simulink model "MC_HEXA_MISSION"  (R2023b)
settings: Solver=FixedStepDiscrete  StartTime=0.0  StopTime=inf  FixedStep=1/250  RelTol=1e-3  EnableMultiTasking=on
values from neighbouring files (symbols this model uses):
  SampleTime = 1/250    (= 0.004)    [Init_FLIGHT_Hexacopter.m]    (also in Init_FLIGHT_Hexacopter_fromNCMS.m = 0.01)
undefined symbols (not defined in the file or in its folder): control, IDLEPWM, MC_PITCH_P, MC_PITCHRATE_D, MC_PITCHRATE_I, MC_PITCHRATE_P, MC_ROLL_P, MC_ROLLRATE_D, MC_ROLLRATE_I, MC_ROLLRATE_P, MC_YAW_P, MC_YAWRATE_D, MC_YAWRATE_I, MC_YAWRATE_P, MPC_XY_P, MPC_XY_VEL_MAX, MPC_Z_D, MPC_Z_I, MPC_Z_P, MPC_Z_VEL_D_ACC, MPC_Z_VEL_I_ACC, MPC_Z_VEL_MAX_DN, MPC_Z_VEL_MAX_UP, MPC_Z_VEL_P_ACC, noutputs, output, pitch, pitch_body, roll, roll_body, TargetHardware, thrust_body, timestamp, x, y, yaw, yaw_body, z
libraries: px4lib x45, px4uORBlib x19, slpidlib x10, simulink x9, px4Utilslib x5, simulink_extras x5, uavalgslib x3, px4Sensorslib x2, sharedutil x1, sharedtransform x1
(part 1 of 4)
settings Model: ExtModeTrigDuration=10  Creator=The MathWorks, Inc.  LastModifiedBy=UASG
settings SolverCC: PositivePriorityOrder=on  MaxZcPerStep=1
settings OptimizationCC: DefaultUnderspecifiedDataType=single  StrengthReduction=on  PassReuseOutputArgsAs=Individual arguments  ZeroExternalMemoryAtStartup=off  ZeroInternalMemoryAtStartup=off  MaxStackSize=64  OptimizeBlockOrder=speed  OptimizationPriority=Speed  OptimizationCustomize=off  MultiThreadedLoops=on  EfficientTunableParamExpr=on
settings DebuggingCC: ParameterTunabilityLossMsg=error
settings HardwareCC: ProdBitPerPointer=32  ProdBitPerSizeT=32  ProdBitPerPtrDiffT=32  ProdLargestAtomicInteger=Long  ProdLargestAtomicFloat=Double  ProdWordSize=32  ProdLongLongMode=on  ProdHWDeviceType=ARM Compatible->ARM Cortex
settings ModelReferenceCC: EnableRefExpFcnMdlSchedulingChecks=on
settings SFSimCC: MATLABDynamicMemAlloc=off  SimTargetLang=C++
settings RTWCC: Description=Embedded Coder  SystemTargetFile=ert.tlc  HardwareBoard=PX4 Cube Orange  TLCOptions="-aInlineSetEventsForThisBaseRateFcn=TLC_FALSE -aSuppressMultiTaskScheduler=TLC_FALSE  -aRateBasedStepFcn=0"  TemplateMakefile=ert_default_tmf  GenerateReport=on  Toolchain=GNU Tools for PX4 Autopilots  BuildConfiguration=Faster Runs  LaunchReport=on  TargetLang=C++  DLArmComputeVersion=19.05
settings CodeAppCC: ForceParamTrailComments=on  IgnoreCustomStorageClasses=off  MaxIdLength=63  OperatorAnnotations=on  SimulinkDataObjDesc=on  SFDataObjDesc=on  InsertBlockDesc=on
settings ERTTargetCC: ExtModeTransport=3  ExtModeStaticAlloc=on  ExtModeStaticAllocSize=1024  ExtModeMexFile=ext_xcp  ExtModeIntrfLevel=Level2 - Open

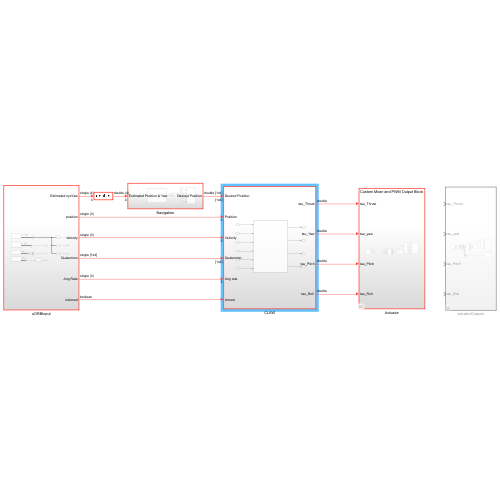
[thumbnail: Simulink's stored preview of the top-level diagram]
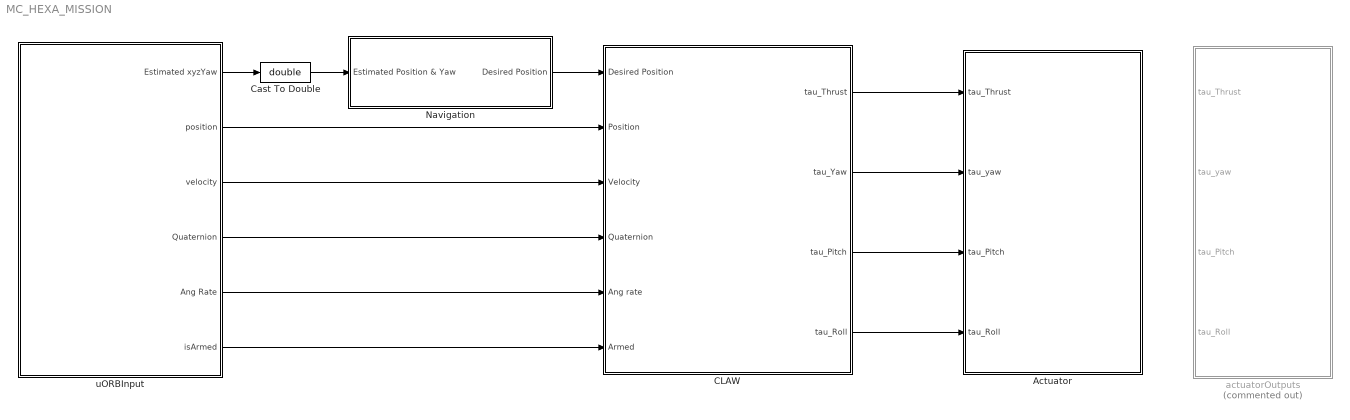
== system MC_HEXA_MISSION ==
  Actuator : Subsystem  Variant=on
  CLAW : Subsystem  RTWFcnName=CLAW
      settings: RTWSystemCode=Nonreusable function  RTWFcnNameOpts=Use subsystem name  RTWFileNameOpts=Use subsystem name
  Cast To Double : DataTypeConversion  OutDataTypeStr=double  SaturateOnIntegerOverflow=off  RndMeth=Floor
  Navigation : Subsystem
      settings: RTWSystemCode=Nonreusable function  RTWFcnNameOpts=Use subsystem name  RTWFileNameOpts=Use subsystem name
  actuatorOutputs : Subsystem  Commented=on  TreatAsAtomicUnit=on
      settings: RTWSystemCode=Nonreusable function  RTWFcnNameOpts=Use subsystem name  RTWFileNameOpts=Use subsystem name
  uORBInput : Subsystem
      settings: RTWSystemCode=Nonreusable function  RTWFcnNameOpts=Use subsystem name  RTWFileNameOpts=Use subsystem name
  wires:
  Navigation/1(Desired Position) -> CLAW/1(Desired Position)
  uORBInput/1(Estimated xyzYaw) -> Cast To Double/1
  uORBInput/3(velocity) -> CLAW/3(Velocity)
  uORBInput/4(Quaternion) -> CLAW/4(Quaternion)
  uORBInput/5(Ang Rate) -> CLAW/5(Ang rate)
  uORBInput/6(isArmed) -> CLAW/6(Armed)
  uORBInput/2(position) -> CLAW/2(Position)
  CLAW/1(tau_Thrust) -> Actuator/1(tau_Thrust)
  CLAW/3(tau_Pitch) -> Actuator/3(tau_Pitch)
  CLAW/2(tau_Yaw) -> Actuator/2(tau_yaw)
  CLAW/4("tau_Roll ") -> Actuator/4(tau_Roll)
  Cast To Double/1 -> Navigation/1(Estimated Position & Yaw)

== system MC_HEXA_MISSION/Actuator ==
  tau_Thrust : Inport
  tau_yaw : Inport  Port=2
  tau_Pitch : Inport  Port=3
  tau_Roll : Inport  Port=4
  Custom Mixer and PWM Output Block : Subsystem  VariantControl=useCustomMixer == true
  PX4 Mixer and actuator_controls_0 topic : Subsystem  VariantControl=useCustomMixer == false

== system MC_HEXA_MISSION/CLAW ==
  Desired Position : Inport
  Position : Inport  Port=2
  Velocity : Inport  Port=3
  Quaternion : Inport  Port=4
  Ang rate : Inport  Port=5
  Armed : Inport  Port=6
  Controller : Subsystem
  tau_Thrust : Outport
  tau_Yaw : Outport  Port=2
  tau_Pitch : Outport  Port=3
  "tau_Roll " : Outport  Port=4
  wires:
  Controller/3(tau_Pitch) -> tau_Pitch/1
  Controller/2(tau_Yaw) -> tau_Yaw/1
  Controller/4("tau_Roll ") -> "tau_Roll "/1
  Controller/1(tau_Thrust) -> tau_Thrust/1
  Desired Position/1 -> Controller/5(Desired Position)
  Position/1 -> Controller/1(Position)
  Velocity/1 -> Controller/2(Velocity)
  Quaternion/1 -> Controller/3(Quaternion)
  Ang rate/1 -> Controller/4(Ang rate)
  Armed/1 -> Controller/6(Armed)

== system MC_HEXA_MISSION/Navigation ==
  Estimated Position & Yaw : Inport
  Demux : Demux
  Quadcopter Navigation Algorithm : Subsystem  Variant=on
  uORB Publish : Subsystem
  Desired Position : Outport
  wires:
  Quadcopter Navigation Algorithm/1(Desired Position) -> Demux/1, Desired Position/1
  Estimated Position & Yaw/1 -> Quadcopter Navigation Algorithm/1(Current Position)
  Demux/1 -> uORB Publish/1(x_sp)
  Demux/2 -> uORB Publish/2(y_sp)
  Demux/3 -> uORB Publish/3(z_sp)
  Demux/4 -> uORB Publish/4(heading_sp)

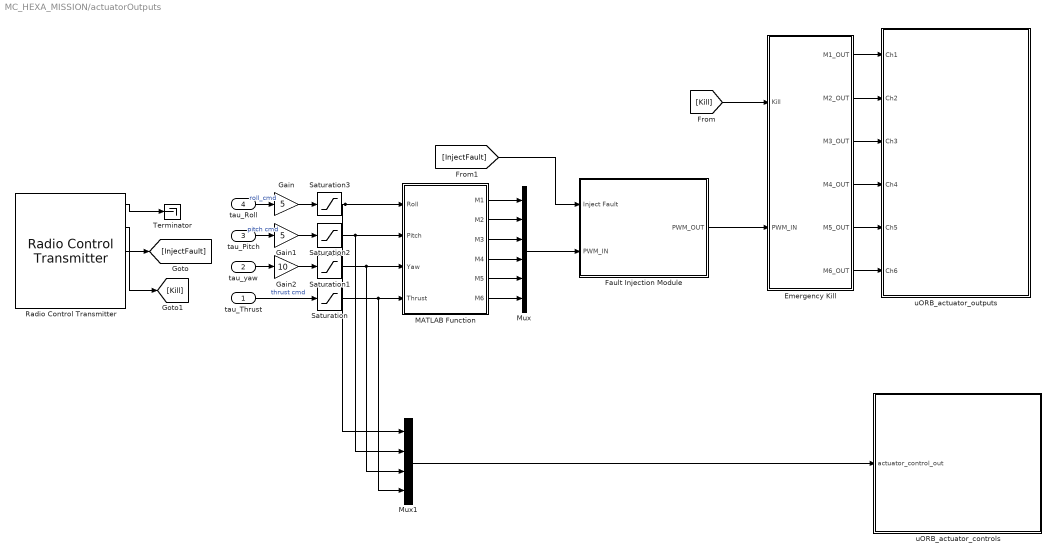
== system MC_HEXA_MISSION/actuatorOutputs ==
  tau_Thrust : Inport
  tau_yaw : Inport  Port=2
  tau_Pitch : Inport  Port=3
  tau_Roll : Inport  Port=4
  Emergency Kill : Subsystem
  Fault Injection Module : Subsystem  Variant=on
  Gain : Gain  Gain=5
  Gain1 : Gain  Gain=5
  Gain2 : Gain  Gain=10
  MATLAB Function : MATLAB Function  TreatAsAtomicUnit=on
  Mux : Mux  Inputs=6
  Mux1 : Mux
  Radio Control Transmitter : px4Sensorslib/Radio Control Transmitter  channel1=off  channel2=off  channel3=off  channel4=off  channel5=off  channel6=on  channel7=on  channel8=off  channel_count=off  rssi=off  rc_input_source=off  timestamp_last_signal=off  time_stamp=off  sampleTime=-1  BlockingMode=off  BlockTimeout=5
  Saturation : Saturate  UpperLimit=1  LowerLimit=0
  Saturation1 : Saturate  UpperLimit=1  LowerLimit=-1
  Saturation2 : Saturate  UpperLimit=1  LowerLimit=-1
  Saturation3 : Saturate  UpperLimit=1  LowerLimit=-1
  Terminator : Terminator
  uORB_actuator_controls : Subsystem
  uORB_actuator_outputs : Subsystem
  wires:
  MATLAB Function/1(M1) -> Mux/1
  Radio Control Transmitter/1 -> Terminator/1
  MATLAB Function/2(M2) -> Mux/2
  tau_Thrust/1 -> Saturation/1  "thrust cmd"
  tau_Pitch/1 -> Gain1/1  "pitch cmd"
  MATLAB Function/3(M3) -> Mux/3
  [Kill] -> Emergency Kill/1(Kill)
  MATLAB Function/6(M6) -> Mux/6
  tau_yaw/1 -> Gain2/1
  Radio Control Transmitter/2 -> [InjectFault]
  Radio Control Transmitter/3 -> [Kill]
  tau_Roll/1 -> Gain/1  "roll_cmd"
  MATLAB Function/4(M4) -> Mux/4
  MATLAB Function/5(M5) -> Mux/5
  [InjectFault] -> Fault Injection Module/1(Inject Fault)
  Mux/1 -> Fault Injection Module/2(PWM_IN)
  Fault Injection Module/1(PWM_OUT) -> Emergency Kill/2(PWM_IN)
  Mux1/1 -> uORB_actuator_controls/1(actuator_control_out)
  Saturation/1 -> Mux1/4, MATLAB Function/4(Thrust)
  Saturation1/1 -> Mux1/3, MATLAB Function/3(Yaw)
  Saturation2/1 -> Mux1/2, MATLAB Function/2(Pitch)
  Saturation3/1 -> Mux1/1, MATLAB Function/1(Roll)
  Gain/1 -> Saturation3/1
  Gain1/1 -> Saturation2/1
  Gain2/1 -> Saturation1/1
  Emergency Kill/1(M1_OUT) -> uORB_actuator_outputs/1(Ch1)
  Emergency Kill/2(M2_OUT) -> uORB_actuator_outputs/2(Ch2)
  Emergency Kill/3(M3_OUT) -> uORB_actuator_outputs/3(Ch3)
  Emergency Kill/4(M4_OUT) -> uORB_actuator_outputs/4(Ch4)
  Emergency Kill/5(M5_OUT) -> uORB_actuator_outputs/5(Ch5)
  Emergency Kill/6(M6_OUT) -> uORB_actuator_outputs/6(Ch6)

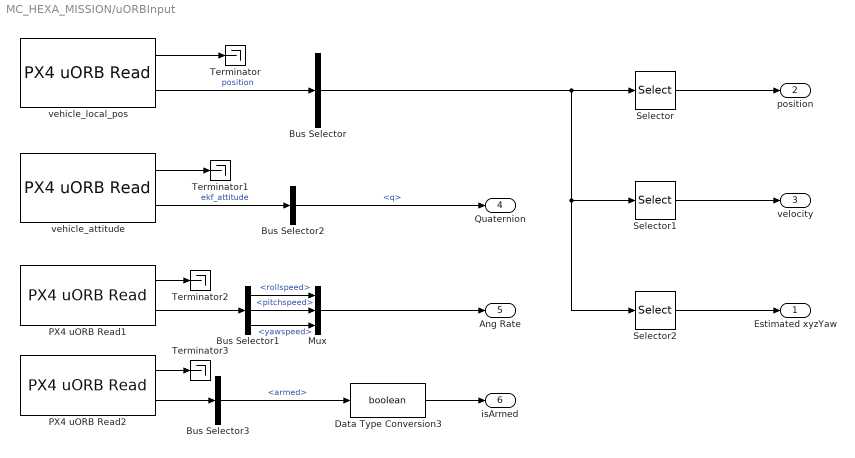
== system MC_HEXA_MISSION/uORBInput ==
  Bus Selector : BusSelector  OutputSignals=x,y,z,vx,vy,vz,heading  OutputAsBus=on
  Bus Selector1 : BusSelector  OutputSignals=rollspeed,pitchspeed,yawspeed
  Bus Selector2 : BusSelector  OutputSignals=q
  Bus Selector3 : BusSelector  OutputSignals=armed
  Data Type Conversion3 : DataTypeConversion  OutDataTypeStr=boolean  SaturateOnIntegerOverflow=off  RndMeth=Floor
  Mux : Mux  Inputs=3
  PX4 uORB Read1 : px4uORBlib/PX4 uORB Read  uORBTopic=vehicle_odometry  selectInstance=vehicle_odometry  SampleTime=-1  BlockingMode=off  BlockTimeout=1e-3
  PX4 uORB Read2 : px4uORBlib/PX4 uORB Read  uORBTopic=actuator_armed  selectInstance=actuator_armed  SampleTime=-1  BlockingMode=off  BlockTimeout=1e-3
  Selector : Selector  InputPortWidth=7  IndexOptions=Index vector (dialog)  Indices=[1:3]  OutputSizes=1
  Selector1 : Selector  InputPortWidth=7  IndexOptions=Index vector (dialog)  Indices=[4:6]  OutputSizes=1
  Selector2 : Selector  InputPortWidth=7  IndexOptions=Index vector (dialog)  Indices=[1 2 3 7]  OutputSizes=1
  Terminator{,1..3} (4 alike) : Terminator
  vehicle_attitude : px4uORBlib/PX4 uORB Read  uORBTopic=vehicle_attitude  selectInstance=vehicle_attitude  SampleTime=-1  BlockingMode=off  BlockTimeout=1e-3
  vehicle_local_pos : px4uORBlib/PX4 uORB Read  uORBTopic=vehicle_local_position  selectInstance=vehicle_local_position  SampleTime=-1  BlockingMode=off  BlockTimeout=1e-3
  Estimated xyzYaw : Outport
  position : Outport  Port=2
  velocity : Outport  Port=3
  Quaternion : Outport  Port=4
  Ang Rate : Outport  Port=5
  isArmed : Outport  Port=6
  wires:
  Bus Selector2/1 -> Quaternion/1  "<q>"
  vehicle_local_pos/2 -> Bus Selector/1  "position"
  Bus Selector/1 -> Selector1/1, Selector2/1, Selector/1
  Selector2/1 -> Estimated xyzYaw/1
  vehicle_attitude/1 -> Terminator1/1
  vehicle_attitude/2 -> Bus Selector2/1  "ekf_attitude"
  vehicle_local_pos/1 -> Terminator/1
  Selector/1 -> position/1
  Selector1/1 -> velocity/1
  PX4 uORB Read1/1 -> Terminator2/1
  Mux/1 -> Ang Rate/1
  PX4 uORB Read1/2 -> Bus Selector1/1
  PX4 uORB Read2/1 -> Terminator3/1
  Bus Selector3/1 -> Data Type Conversion3/1  "<armed>"
  PX4 uORB Read2/2 -> Bus Selector3/1
  Bus Selector1/1 -> Mux/1  "<rollspeed>"
  Bus Selector1/2 -> Mux/2  "<pitchspeed>"
  Bus Selector1/3 -> Mux/3  "<yawspeed>"
  Data Type Conversion3/1 -> isArmed/1

== system MC_HEXA_MISSION/Actuator/Custom Mixer and PWM Output Block ==
  tau_Thrust : Inport
  tau_yaw : Inport  Port=2
  tau_Pitch : Inport  Port=3
  tau_Roll : Inport  Port=4
  Emergency Kill : Subsystem
  Fault_Injection : Subsystem
      settings: PortSchema="{\"entries\":[{\"content\":{\"sides\":[{\"content\":{\"connectorIds\":[\"In1\"]},\"type\":\"ConnectorPlacement.EquallySpacedRectSide\",\"uuid\":\"fab26c65-8d77-46b7-b375-2033d08e8306\"},{\"content\":{\"connectorIds\":[\"Out1\"],\"side\":\"RIGHT\"},\"type\":\"ConnectorPlacement.EquallySpacedRectSide\",\"uuid\":\"bc3f50bd-e170-4b75-8089-4f92da68e83e\"},{\"content\":{\"connectorIds\":[\"In2\"],\"side\":\"TOP\"},\"type\":\"ConnectorPlacement.EquallySpacedRectSide\",\"uuid\":\"873ada90-6f93-48ab-a701-a52d28357753\"}]},\"type\":\"ConnectorPlacement.EquallySpacedConnector\",\"uuid\":\"201be8b3-bff4-4924-8e0c-28e5fee33d1c\"}],\"packageUris\":[\"http://schema.mathworks.com/mf0/Connector/R2020b\"],\"version\":\"1.0\"}"
  Gain : Gain  Gain=5
  Gain1 : Gain  Gain=5
  Gain2 : Gain  Gain=10
  Gain3 : Gain
  MATLAB Function : MATLAB Function  TreatAsAtomicUnit=on
  Mux : Mux  Inputs=6
  Radio Control Transmitter : px4Sensorslib/Radio Control Transmitter  channel1=off  channel2=off  channel3=off  channel4=off  channel5=off  channel6=off  channel7=on  channel8=on  channel_count=off  rssi=off  rc_input_source=off  timestamp_last_signal=off  time_stamp=off  sampleTime=-1  BlockingMode=off  BlockTimeout=5
  Subsystem : Subsystem
  Terminator : Terminator
  wires:
  Radio Control Transmitter/2 -> [Kill]
  [InjectFault] -> Fault_Injection/2(Inject Fault)
  Fault_Injection/1(PWM_OUT) -> Emergency Kill/2(PWM_IN)
  [Kill] -> Emergency Kill/1(Kill)
  Radio Control Transmitter/3 -> [InjectFault]
  Radio Control Transmitter/1 -> Terminator/1
  Emergency Kill/2(M2_OUT) -> Subsystem/2(Ch2)
  Emergency Kill/3(M3_OUT) -> Subsystem/3(Ch3)
  Emergency Kill/4(M4_OUT) -> Subsystem/4(Ch4)
  Emergency Kill/5(M5_OUT) -> Subsystem/5(Ch5)
  Emergency Kill/6(M6_OUT) -> Subsystem/6(Ch6)
  Emergency Kill/1(M1_OUT) -> Subsystem/1(Ch1)
  tau_Thrust/1 -> Gain3/1  "thrust cmd"
  tau_Roll/1 -> Gain/1  "roll_cmd"
  tau_Pitch/1 -> Gain1/1  "pitch cmd"
  tau_yaw/1 -> Gain2/1
  MATLAB Function/1(M1) -> Mux/1
  MATLAB Function/2(M2) -> Mux/2
  MATLAB Function/3(M3) -> Mux/3
  MATLAB Function/4(M4) -> Mux/4
  MATLAB Function/5(M5) -> Mux/5
  MATLAB Function/6(M6) -> Mux/6
  Mux/1 -> Fault_Injection/1(PWM_IN)
  Gain/1 -> MATLAB Function/1(Roll)
  Gain1/1 -> MATLAB Function/2(Pitch)
  Gain2/1 -> MATLAB Function/3(Yaw)
  Gain3/1 -> MATLAB Function/4(Thrust)

== system MC_HEXA_MISSION/Actuator/PX4 Mixer and actuator_controls_0 topic ==
  tau_Thrust : Inport
  tau_yaw : Inport  Port=2
  tau_Pitch : Inport  Port=3
  tau_Roll : Inport  Port=4
  Armed : Inport  Port=5
  Bus Assignment : BusAssignment  AssignedSignals=control
  Constant : Constant  Value=zeros(4,1)
  Data Type Conversion : DataTypeConversion  SaturateOnIntegerOverflow=off  RndMeth=Floor
  Mux : Mux  Inputs=5
  PX4 uORB Message : px4uORBlib/PX4 uORB Message  uORBTopic=actuator_controls  SampleTime=inf  selectInstance=vehicle_gps_position
  PX4 uORB Write : px4uORBlib/PX4 uORB Write  uORBTopic=actuator_controls  selectInstance=actuator_controls_0  MessageQueueLen=1
  Terminator : Terminator
  wires:
  Bus Assignment/1 -> PX4 uORB Write/1
  tau_yaw/1 -> Mux/3
  Data Type Conversion/1 -> Bus Assignment/2
  tau_Roll/1 -> Mux/1  "roll_cmd"
  PX4 uORB Message/1 -> Bus Assignment/1
  Mux/1 -> Data Type Conversion/1
  Constant/1 -> Mux/5
  tau_Pitch/1 -> Mux/2  "pitch cmd"
  tau_Thrust/1 -> Mux/4  "thrust cmd"
  Armed/1 -> Terminator/1

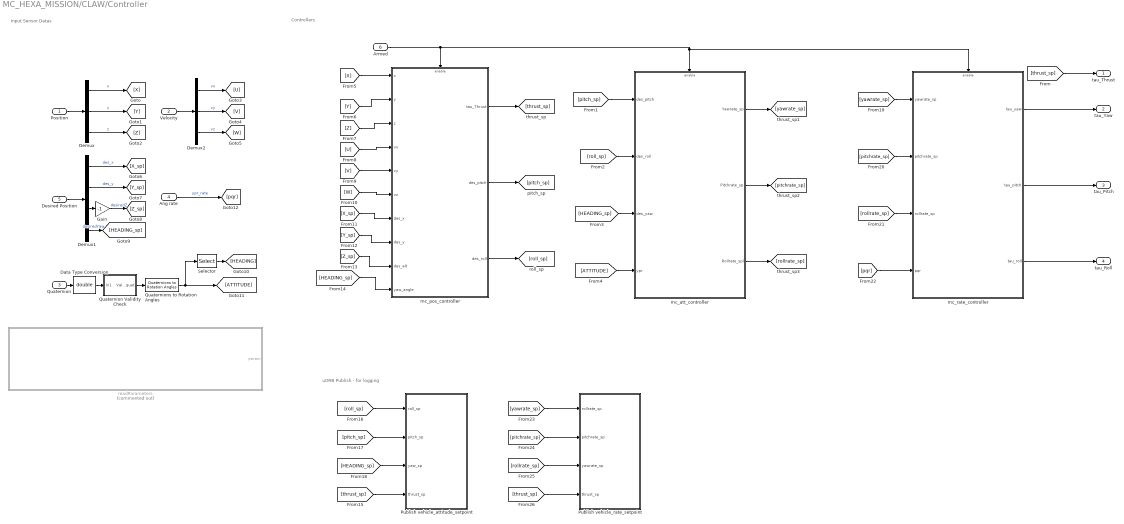
== system MC_HEXA_MISSION/CLAW/Controller ==
  note: uORB Publish - for logging
  note: Controllers
  note: Input Sensor Datas
  Position : Inport
  Velocity : Inport  Port=2
  Quaternion : Inport  Port=3
  Ang rate : Inport  Port=4
  Desired Position : Inport  Port=5
  Armed : Inport  Port=6
  Data Type Conversion : DataTypeConversion  OutDataTypeStr=double  SaturateOnIntegerOverflow=off  RndMeth=Floor
  Demux : Demux  Outputs=3
  Demux1 : Demux
  Demux2 : Demux  Outputs=3
  Gain : Gain  Gain=-1
  Publish vehicle_attitude_setpoint : Subsystem
  Publish vehicle_rate_setpoint : Subsystem
  Quaternion Validity Check : Subsystem
  Quaternions to Rotation Angles : sharedtransform/Quaternions to Rotation Angles  rotationOrder=ZYX  aMode=aMode
  Selector : Selector  InputPortWidth=3  IndexOptions=Index vector (dialog)  Indices=[1]  OutputSizes=1
  mc_att_controller : Subsystem
      settings: RTWSystemCode=Nonreusable function  RTWFcnNameOpts=Use subsystem name  RTWFileNameOpts=Use subsystem name
  mc_pos_controller : Subsystem
      settings: RTWSystemCode=Nonreusable function  RTWFcnNameOpts=Use subsystem name  RTWFileNameOpts=Use subsystem name
  mc_rate_controller : Subsystem
      settings: RTWSystemCode=Nonreusable function  RTWFcnNameOpts=Use subsystem name  RTWFileNameOpts=Use subsystem name
  readParameters : Subsystem  Commented=on  TreatAsAtomicUnit=on
  tau_Thrust : Outport
  tau_Yaw : Outport  Port=2
  tau_Pitch : Outport  Port=3
  "tau_Roll " : Outport  Port=4
  wires:
  Demux1/3 -> Gain/1
  Desired Position/1 -> Demux1/1
  Quaternion/1 -> Data Type Conversion/1
  Data Type Conversion/1 -> Quaternion Validity Check/1(In1)
  Position/1 -> Demux/1
  Velocity/1 -> Demux2/1
  Quaternion Validity Check/1(Valid quat) -> Quaternions to Rotation Angles/1
  Quaternions to Rotation Angles/1 -> [ATTITUDE], Selector/1
  mc_pos_controller/1(tau_Thrust) -> [thrust_sp]
  mc_pos_controller/2(des_pitch) -> [pitch_sp]
  mc_pos_controller/3(des_roll) -> [roll_sp]
  Demux/3 -> [Z]  "z"
  Demux/2 -> [Y]  "y"
  Demux/1 -> [X]  "x"
  Demux2/2 -> [V]  "vy"
  Demux2/1 -> [U]  "vx"
  Demux2/3 -> [W]  "vz"
  Demux1/1 -> [X_sp]  "des_x"
  Demux1/2 -> [Y_sp]  "des_y"
  Gain/1 -> [Z_sp]  "desiredZ"
  Demux1/4 -> [HEADING_sp]  "desiredYaw"
  Selector/1 -> [HEADING]
  [thrust_sp] -> tau_Thrust/1
  [roll_sp] -> mc_att_controller/2(des_roll)
  [pitch_sp] -> mc_att_controller/1(des_pitch)
  [HEADING_sp] -> mc_att_controller/3(des_yaw)
  [ATTITUDE] -> mc_att_controller/4(ypr)
  [X] -> mc_pos_controller/1(x)
  [Y] -> mc_pos_controller/2(y)
  [Z] -> mc_pos_controller/3(z)
  [U] -> mc_pos_controller/4(vx)
  [V] -> mc_pos_controller/5(vy)
  [W] -> mc_pos_controller/6(vz)
  [X_sp] -> mc_pos_controller/7(des_x)
  [Y_sp] -> mc_pos_controller/8(des_y)
  [Z_sp] -> mc_pos_controller/9(des_alt)
  [HEADING_sp] -> mc_pos_controller/10(yaw_angle)
  [thrust_sp] -> Publish vehicle_attitude_setpoint/4(thrust_sp)
  [roll_sp] -> Publish vehicle_attitude_setpoint/1(roll_sp)
  [pitch_sp] -> Publish vehicle_attitude_setpoint/2(pitch_sp)
  [HEADING_sp] -> Publish vehicle_attitude_setpoint/3(yaw_sp)
  Ang rate/1 -> [pqr]  "ypr_rate"
  mc_att_controller/1(Yawrate_sp) -> [yawrate_sp]
  mc_att_controller/2(Pitchrate_sp) -> [pitchrate_sp]
  mc_att_controller/3(Rollrate_spl) -> [rollrate_sp]
  [yawrate_sp] -> mc_rate_controller/1(yawrate_sp)
  [pitchrate_sp] -> mc_rate_controller/2(pitchrate_sp)
  [rollrate_sp] -> mc_rate_controller/3(rollrate_sp)
  mc_rate_controller/1(tau_yaw) -> tau_Yaw/1
  mc_rate_controller/2(tau_pitch) -> tau_Pitch/1
  mc_rate_controller/3(tau_roll) -> "tau_Roll "/1
  [pqr] -> mc_rate_controller/4(pqr)
  [yawrate_sp] -> Publish vehicle_rate_setpoint/1(rollrate_sp)
  [thrust_sp] -> Publish vehicle_rate_setpoint/4(thrust_sp)
  [pitchrate_sp] -> Publish vehicle_rate_setpoint/2(pitchrate_sp)
  [rollrate_sp] -> Publish vehicle_rate_setpoint/3(yawrate_sp)
  Armed/1 -> mc_rate_controller/Enable, mc_att_controller/Enable, mc_pos_controller/Enable

== system MC_HEXA_MISSION/Navigation/Quadcopter Navigation Algorithm ==
  Current Position : Inport
  Manual Waypoints : Subsystem  VariantControl=guidanceType == 3
  Manual Waypoints from Simulink Dashboard : Subsystem  VariantControl=guidanceType == 2
  Path Correction from Onboard Computer : Subsystem  VariantControl=guidanceType == 1
  Read waypoint from QGroundControl Mission : Subsystem  VariantControl=guidanceType == 0
  Desired Position : Outport

== system MC_HEXA_MISSION/Navigation/uORB Publish ==
  x_sp : Inport
  y_sp : Inport  Port=2
  z_sp : Inport  Port=3
  heading_sp : Inport  Port=4
  Bus Assignment : BusAssignment  AssignedSignals=timestamp,x,y,z,yaw
  Data Type Conversion{,1..3} (4 alike) : DataTypeConversion  OutDataTypeStr=single  SaturateOnIntegerOverflow=off  RndMeth=Floor
  PX4 Timestamp : px4Utilslib/PX4 Timestamp  SampleTime=-1
  PX4 uORB Message : px4uORBlib/PX4 uORB Message  uORBTopic=vehicle_local_position_setpoint  SampleTime=-1  selectInstance=actuator_controls
  PX4 uORB Write : px4uORBlib/PX4 uORB Write  uORBTopic=vehicle_local_position_setpoint  selectInstance=vehicle_local_position_setpoint  MessageQueueLen=1
  wires:
  PX4 Timestamp/1 -> Bus Assignment/2
  Bus Assignment/1 -> PX4 uORB Write/1
  PX4 uORB Message/1 -> Bus Assignment/1
  x_sp/1 -> Data Type Conversion/1
  y_sp/1 -> Data Type Conversion1/1
  z_sp/1 -> Data Type Conversion2/1
  Data Type Conversion/1 -> Bus Assignment/3
  Data Type Conversion1/1 -> Bus Assignment/4
  Data Type Conversion2/1 -> Bus Assignment/5
  Data Type Conversion3/1 -> Bus Assignment/6
  heading_sp/1 -> Data Type Conversion3/1

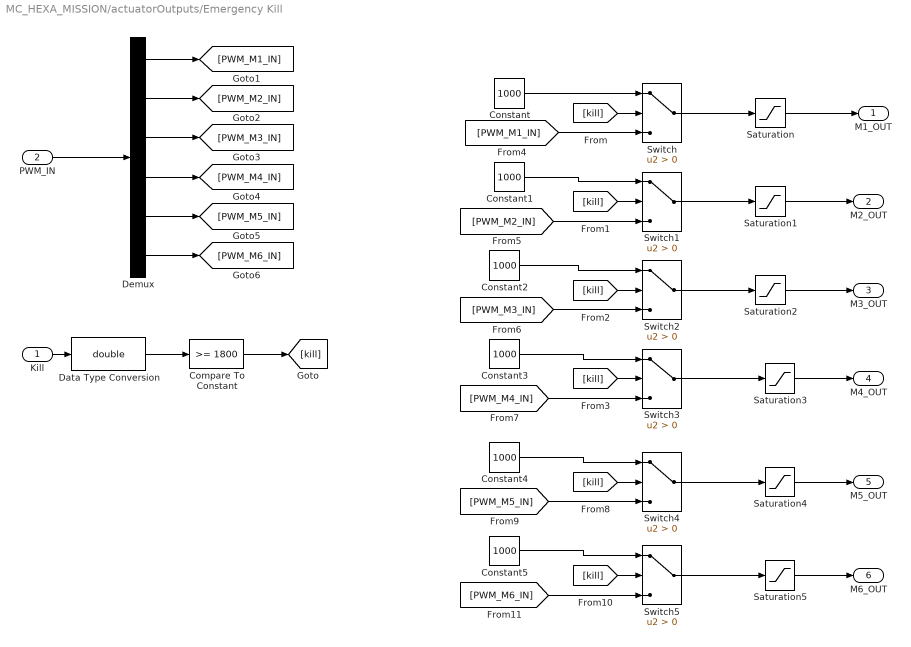
== system MC_HEXA_MISSION/actuatorOutputs/Emergency Kill ==
  Kill : Inport
  PWM_IN : Inport  Port=2
  Compare To Constant : simulink/Logic and Bit Operations/Compare To Constant  relop=>=  const=1800  OutDataTypeStr=boolean
  Constant{,1..5} (6 alike) : Constant  Value=1000
  Data Type Conversion : DataTypeConversion  OutDataTypeStr=double  SaturateOnIntegerOverflow=off  RndMeth=Floor
  Demux : Demux  Outputs=6
  Saturation{,1..5} (6 alike) : Saturate  UpperLimit=2000  LowerLimit=900
  Switch{,1..5} (6 alike) : Switch  Criteria=u2 > Threshold  SaturateOnIntegerOverflow=off  InputSameDT=off
  M1_OUT : Outport
  M2_OUT : Outport  Port=2
  M3_OUT : Outport  Port=3
  M4_OUT : Outport  Port=4
  M5_OUT : Outport  Port=5
  M6_OUT : Outport  Port=6
  wires:
  Kill/1 -> Data Type Conversion/1
  Data Type Conversion/1 -> Compare To Constant/1
  Compare To Constant/1 -> [kill]
  [kill] -> Switch/2
  Constant/1 -> Switch/1
  [kill] -> Switch1/2
  [kill] -> Switch2/2
  [kill] -> Switch3/2
  [PWM_M2_IN] -> Switch1/3
  Constant1/1 -> Switch1/1
  [PWM_M3_IN] -> Switch2/3
  Constant2/1 -> Switch2/1
  [PWM_M4_IN] -> Switch3/3
  Constant3/1 -> Switch3/1
  Switch/1 -> Saturation/1
  Switch1/1 -> Saturation1/1
  Switch2/1 -> Saturation2/1
  Switch3/1 -> Saturation3/1
  PWM_IN/1 -> Demux/1
  Demux/1 -> [PWM_M1_IN]
  Demux/2 -> [PWM_M2_IN]
  Demux/3 -> [PWM_M3_IN]
  Demux/4 -> [PWM_M4_IN]
  [PWM_M1_IN] -> Switch/3
  Demux/5 -> [PWM_M5_IN]
  Demux/6 -> [PWM_M6_IN]
  Constant4/1 -> Switch4/1
  [PWM_M5_IN] -> Switch4/3
  [kill] -> Switch4/2
  Switch4/1 -> Saturation4/1
  Constant5/1 -> Switch5/1
  [PWM_M6_IN] -> Switch5/3
  [kill] -> Switch5/2
  Switch5/1 -> Saturation5/1
  Saturation/1 -> M1_OUT/1
  Saturation1/1 -> M2_OUT/1
  Saturation2/1 -> M3_OUT/1
  Saturation3/1 -> M4_OUT/1
  Saturation4/1 -> M5_OUT/1
  Saturation5/1 -> M6_OUT/1

== system MC_HEXA_MISSION/actuatorOutputs/Fault Injection Module ==
  Inject Fault : Inport
  PWM_IN : Inport  Port=2
  Fault_Injection : Subsystem  VariantControl=(default)
      settings: PortSchema="{\"entries\":[{\"content\":{\"sides\":[{\"content\":{\"connectorIds\":[\"In1\"]},\"type\":\"ConnectorPlacement.EquallySpacedRectSide\",\"uuid\":\"fab26c65-8d77-46b7-b375-2033d08e8306\"},{\"content\":{\"connectorIds\":[\"Out1\"],\"side\":\"RIGHT\"},\"type\":\"ConnectorPlacement.EquallySpacedRectSide\",\"uuid\":\"bc3f50bd-e170-4b75-8089-4f92da68e83e\"},{\"content\":{\"connectorIds\":[\"In2\"],\"side\":\"TOP\"},\"type\":\"ConnectorPlacement.EquallySpacedRectSide\",\"uuid\":\"873ada90-6f93-48ab-a701-a52d28357753\"}]},\"type\":\"ConnectorPlacement.EquallySpacedConnector\",\"uuid\":\"201be8b3-bff4-4924-8e0c-28e5fee33d1c\"}],\"packageUris\":[\"http://schema.mathworks.com/mf0/Connector/R2020b\"],\"version\":\"1.0\"}"
  Fault_Injection_SIL : Subsystem  VariantControl="strcmp(TargetHardware,\"SITL\")"
      settings: PortSchema="{\"entries\":[{\"content\":{\"sides\":[{\"content\":{\"connectorIds\":[\"In1\"]},\"type\":\"ConnectorPlacement.EquallySpacedRectSide\",\"uuid\":\"fab26c65-8d77-46b7-b375-2033d08e8306\"},{\"content\":{\"connectorIds\":[\"Out1\"],\"side\":\"RIGHT\"},\"type\":\"ConnectorPlacement.EquallySpacedRectSide\",\"uuid\":\"bc3f50bd-e170-4b75-8089-4f92da68e83e\"},{\"content\":{\"connectorIds\":[\"In2\"],\"side\":\"TOP\"},\"type\":\"ConnectorPlacement.EquallySpacedRectSide\",\"uuid\":\"873ada90-6f93-48ab-a701-a52d28357753\"}]},\"type\":\"ConnectorPlacement.EquallySpacedConnector\",\"uuid\":\"201be8b3-bff4-4924-8e0c-28e5fee33d1c\"}],\"packageUris\":[\"http://schema.mathworks.com/mf0/Connector/R2020b\"],\"version\":\"1.0\"}"
  PWM_OUT : Outport

== system MC_HEXA_MISSION/actuatorOutputs/uORB_actuator_controls ==
  actuator_control_out : Inport
  Bus Assignment : BusAssignment  AssignedSignals=timestamp,control
  Constant : Constant  Value=0
  Data Type 1 : DataTypeConversion  OutDataTypeStr=single  RndMeth=Floor
  Data Type 7 : DataTypeConversion  OutDataTypeStr=single  RndMeth=Floor
  Demux : Demux
  Mux : Mux  Inputs=8
  PX4 Timestamp : px4Utilslib/PX4 Timestamp  SampleTime=-1
  PX4 uORB Message : px4uORBlib/PX4 uORB Message  uORBTopic=actuator_controls  SampleTime=-1  selectInstance=actuator_controls
  PX4 uORB Write : px4uORBlib/PX4 uORB Write  uORBTopic=actuator_controls  selectInstance=actuator_controls_0  MessageQueueLen=1
  wires:
  Bus Assignment/1 -> PX4 uORB Write/1
  PX4 uORB Message/1 -> Bus Assignment/1
  actuator_control_out/1 -> Data Type 7/1
  Mux/1 -> Bus Assignment/3
  Data Type 7/1 -> Demux/1
  Demux/1 -> Mux/1
  Demux/2 -> Mux/2
  Demux/3 -> Mux/3
  Demux/4 -> Mux/4
  Constant/1 -> Data Type 1/1
  Data Type 1/1 -> Mux/8, Mux/7, Mux/6, Mux/5
  PX4 Timestamp/1 -> Bus Assignment/2

== system MC_HEXA_MISSION/actuatorOutputs/uORB_actuator_outputs ==
  Ch1 : Inport
  Ch2 : Inport  Port=2
  Ch3 : Inport  Port=3
  Ch4 : Inport  Port=4
  Ch5 : Inport  Port=5
  Ch6 : Inport  Port=6
  Bus Assignment : BusAssignment  AssignedSignals=timestamp,noutputs,output
  Constant : Constant  Value=0
  Constant17 : Constant  Value=6  OutDataTypeStr=uint32
  Data Type Conversion : DataTypeConversion  OutDataTypeStr=single  SaturateOnIntegerOverflow=off  RndMeth=Floor
  Data Type Conversion1 : DataTypeConversion  OutDataTypeStr=uint32  SaturateOnIntegerOverflow=off  RndMeth=Floor
  Mux1 : Mux  Inputs=16
  PX4 Timestamp1 : px4Utilslib/PX4 Timestamp  SampleTime=-1
  PX4 uORB Message : px4uORBlib/PX4 uORB Message  uORBTopic=actuator_outputs  SampleTime=-1  selectInstance=actuator_outputs
  PX4 uORB Write : px4uORBlib/PX4 uORB Write  uORBTopic=actuator_outputs  selectInstance=actuator_outputs  MessageQueueLen=1
  wires:
  Data Type Conversion1/1 -> Bus Assignment/3
  PX4 Timestamp1/1 -> Bus Assignment/2
  Bus Assignment/1 -> PX4 uORB Write/1
  PX4 uORB Message/1 -> Bus Assignment/1
  Mux1/1 -> Data Type Conversion/1
  Constant17/1 -> Data Type Conversion1/1
  Data Type Conversion/1 -> Bus Assignment/4
  Ch1/1 -> Mux1/1
  Ch2/1 -> Mux1/2
  Ch3/1 -> Mux1/3
  Ch4/1 -> Mux1/4
  Ch5/1 -> Mux1/5
  Constant/1 -> Mux1/11, Mux1/12, Mux1/13, Mux1/14, Mux1/16, Mux1/15, Mux1/10, Mux1/9, Mux1/8, Mux1/7
  Ch6/1 -> Mux1/6

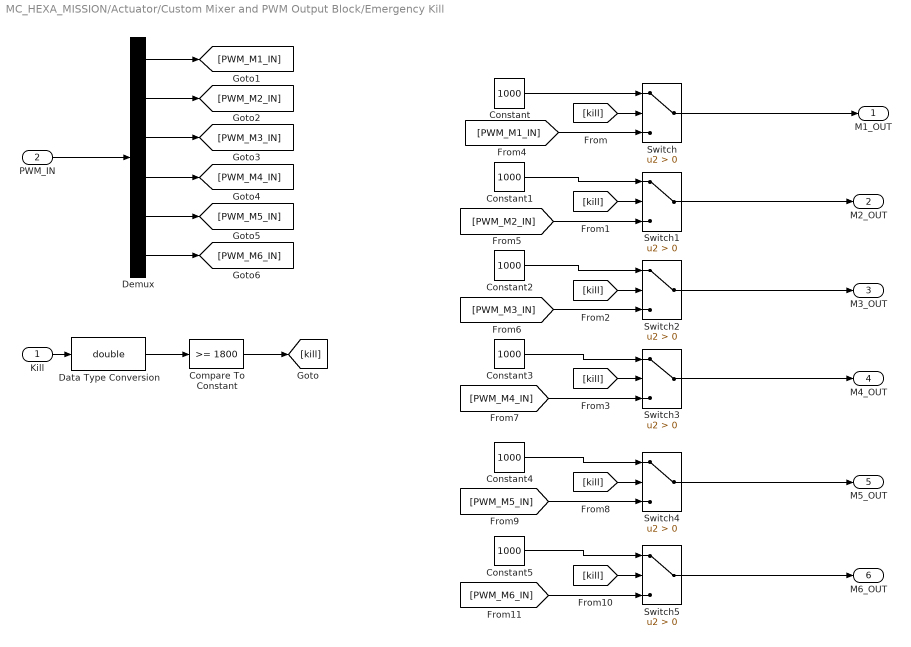
== system MC_HEXA_MISSION/Actuator/Custom Mixer and PWM Output Block/Emergency Kill ==
  Kill : Inport
  PWM_IN : Inport  Port=2
  Compare To Constant : simulink/Logic and Bit Operations/Compare To Constant  relop=>=  const=1800  OutDataTypeStr=boolean
  Constant{,1..5} (6 alike) : Constant  Value=1000
  Data Type Conversion : DataTypeConversion  OutDataTypeStr=double  SaturateOnIntegerOverflow=off  RndMeth=Floor
  Demux : Demux  Outputs=6
  Switch{,1..5} (6 alike) : Switch  Criteria=u2 > Threshold  SaturateOnIntegerOverflow=off  InputSameDT=off
  M1_OUT : Outport
  M2_OUT : Outport  Port=2
  M3_OUT : Outport  Port=3
  M4_OUT : Outport  Port=4
  M5_OUT : Outport  Port=5
  M6_OUT : Outport  Port=6
  wires:
  Kill/1 -> Data Type Conversion/1
  Data Type Conversion/1 -> Compare To Constant/1
  Compare To Constant/1 -> [kill]
  [kill] -> Switch/2
  Constant/1 -> Switch/1
  [kill] -> Switch1/2
  [kill] -> Switch2/2
  [kill] -> Switch3/2
  [PWM_M2_IN] -> Switch1/3
  Constant1/1 -> Switch1/1
  [PWM_M3_IN] -> Switch2/3
  Constant2/1 -> Switch2/1
  [PWM_M4_IN] -> Switch3/3
  Constant3/1 -> Switch3/1
  Switch/1 -> M1_OUT/1
  Switch1/1 -> M2_OUT/1
  Switch2/1 -> M3_OUT/1
  Switch3/1 -> M4_OUT/1
  PWM_IN/1 -> Demux/1
  Demux/1 -> [PWM_M1_IN]
  Demux/2 -> [PWM_M2_IN]
  Demux/3 -> [PWM_M3_IN]
  Demux/4 -> [PWM_M4_IN]
  [PWM_M1_IN] -> Switch/3
  Demux/5 -> [PWM_M5_IN]
  Demux/6 -> [PWM_M6_IN]
  Constant4/1 -> Switch4/1
  [PWM_M5_IN] -> Switch4/3
  [kill] -> Switch4/2
  Switch4/1 -> M5_OUT/1
  Constant5/1 -> Switch5/1
  [PWM_M6_IN] -> Switch5/3
  [kill] -> Switch5/2
  Switch5/1 -> M6_OUT/1

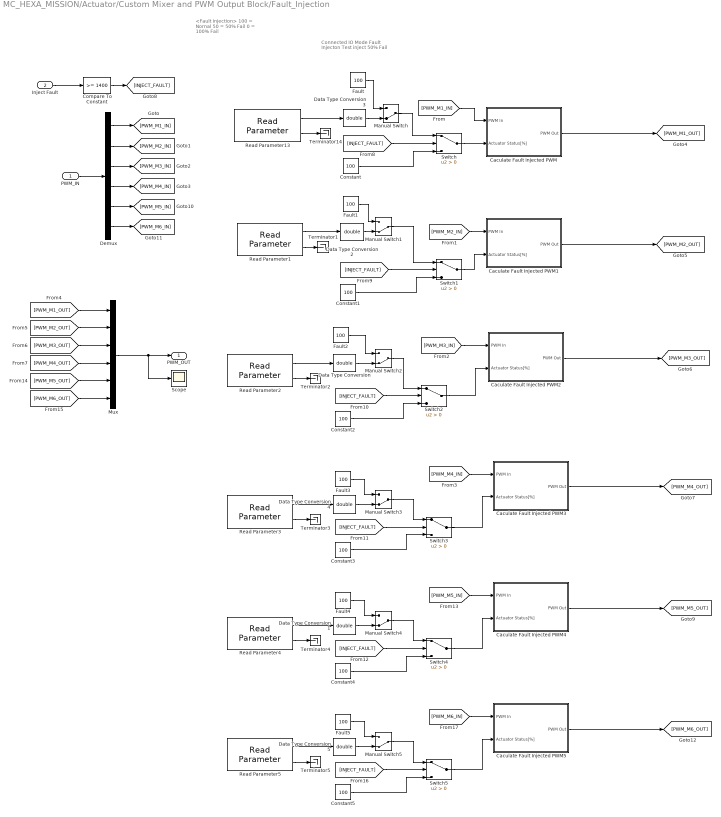
== system MC_HEXA_MISSION/Actuator/Custom Mixer and PWM Output Block/Fault_Injection ==
  note: Connected IO Mode
      | Fault Injecton Test
      |
      | inject 50% Fail
  note: <Fault Injection>
      | 100 = Nornal
      | 50 = 50% Fail
      | 0 = 100% Fail
  PWM_IN : Inport
  Inject Fault : Inport  Port=2
  Caculate Fault Injected PWM : Subsystem
  Caculate Fault Injected PWM1 : Subsystem
  Caculate Fault Injected PWM2 : Subsystem
  Caculate Fault Injected PWM3 : Subsystem
  Caculate Fault Injected PWM4 : Subsystem
  Caculate Fault Injected PWM5 : Subsystem
  Compare To Constant : simulink/Logic and Bit Operations/Compare To Constant  relop=>=  const=1400  OutDataTypeStr=boolean
  Constant{,1..5} (6 alike) : Constant  Value=100
  Data Type Conversion{,1..5} (6 alike) : DataTypeConversion  OutDataTypeStr=double  SaturateOnIntegerOverflow=off  RndMeth=Floor
  Demux : Demux  Outputs=6
  Fault{,1..5} (6 alike) : Constant  Value=100
  Manual Switch{,1..5} (6 alike) : ManualSwitch  CurrentSetting=0
  Mux : Mux  Inputs=6
  Read Parameter1 : px4lib/Read Parameter  ParameterName=FDD_M2_STATUS  DataType=INT32  SampleTime=-1
  Read Parameter13 : px4lib/Read Parameter  ParameterName=FDD_M1_STATUS  DataType=INT32  SampleTime=-1
  Read Parameter2 : px4lib/Read Parameter  ParameterName=FDD_M3_STATUS  DataType=INT32  SampleTime=-1
  Read Parameter3 : px4lib/Read Parameter  ParameterName=FDD_M4_STATUS  DataType=INT32  SampleTime=-1
  Read Parameter4 : px4lib/Read Parameter  ParameterName=FDD_M5_STATUS  DataType=INT32  SampleTime=-1
  Read Parameter5 : px4lib/Read Parameter  ParameterName=FDD_M6_STATUS  DataType=INT32  SampleTime=-1
  Scope : Scope
  Switch{,1..5} (6 alike) : Switch  Criteria=u2 > Threshold  SaturateOnIntegerOverflow=off  InputSameDT=off
  Terminator{1..5,14} (6 alike) : Terminator
  PWM_OUT : Outport
  wires:
  Read Parameter13/2 -> Terminator14/1
  Read Parameter1/2 -> Terminator1/1
  Read Parameter2/2 -> Terminator2/1
  Read Parameter2/1 -> Data Type Conversion/1
  Read Parameter3/2 -> Terminator3/1
  Read Parameter3/1 -> Data Type Conversion4/1
  Data Type Conversion/1 -> Manual Switch2/2
  Data Type Conversion4/1 -> Manual Switch3/2
  Read Parameter13/1 -> Data Type Conversion3/1
  Read Parameter1/1 -> Data Type Conversion2/1
  Data Type Conversion3/1 -> Manual Switch/2
  Fault/1 -> Manual Switch/1
  Data Type Conversion2/1 -> Manual Switch1/2
  Fault1/1 -> Manual Switch1/1
  Fault2/1 -> Manual Switch2/1
  Fault3/1 -> Manual Switch3/1
  PWM_IN/1 -> Demux/1
  Demux/1 -> [PWM_M1_IN]
  Demux/2 -> [PWM_M2_IN]
  Demux/3 -> [PWM_M3_IN]
  Demux/4 -> [PWM_M4_IN]
  [PWM_M1_IN] -> Caculate Fault Injected PWM/1(PWM In)
  [PWM_M2_IN] -> Caculate Fault Injected PWM1/1(PWM In)
  [PWM_M3_IN] -> Caculate Fault Injected PWM2/1(PWM In)
  [PWM_M4_IN] -> Caculate Fault Injected PWM3/1(PWM In)
  Mux/1 -> Scope/1, PWM_OUT/1
  [PWM_M1_OUT] -> Mux/1
  [PWM_M2_OUT] -> Mux/2
  [PWM_M3_OUT] -> Mux/3
  [PWM_M4_OUT] -> Mux/4
  Inject Fault/1 -> Compare To Constant/1
  Compare To Constant/1 -> [INJECT_FAULT]
  Manual Switch/1 -> Switch/1
  Switch/1 -> Caculate Fault Injected PWM/2(" Actuator Status[%]")
  [INJECT_FAULT] -> Switch/2
  Constant/1 -> Switch/3
  Constant1/1 -> Switch1/3
  [INJECT_FAULT] -> Switch1/2
  Switch1/1 -> Caculate Fault Injected PWM1/2(" Actuator Status[%]")
  Manual Switch1/1 -> Switch1/1
  Switch2/1 -> Caculate Fault Injected PWM2/2(" Actuator Status[%]")
  Constant2/1 -> Switch2/3
  [INJECT_FAULT] -> Switch2/2
  Manual Switch2/1 -> Switch2/1
  Switch3/1 -> Caculate Fault Injected PWM3/2(" Actuator Status[%]")
  Constant3/1 -> Switch3/3
  [INJECT_FAULT] -> Switch3/2
  Manual Switch3/1 -> Switch3/1
  [PWM_M5_IN] -> Caculate Fault Injected PWM4/1(PWM In)
  Read Parameter4/1 -> Data Type Conversion1/1
  Fault4/1 -> Manual Switch4/1
  Switch4/1 -> Caculate Fault Injected PWM4/2(" Actuator Status[%]")
  Manual Switch4/1 -> Switch4/1
  Constant4/1 -> Switch4/3
  Data Type Conversion1/1 -> Manual Switch4/2
  Read Parameter4/2 -> Terminator4/1
  [INJECT_FAULT] -> Switch4/2
  Demux/5 -> [PWM_M5_IN]
  Demux/6 -> [PWM_M6_IN]
  [PWM_M5_OUT] -> Mux/5
  [PWM_M6_OUT] -> Mux/6
  Fault5/1 -> Manual Switch5/1
  [PWM_M6_IN] -> Caculate Fault Injected PWM5/1(PWM In)
  Manual Switch5/1 -> Switch5/1
  Read Parameter5/2 -> Terminator5/1
  [INJECT_FAULT] -> Switch5/2
  Read Parameter5/1 -> Data Type Conversion5/1
  Constant5/1 -> Switch5/3
  Data Type Conversion5/1 -> Manual Switch5/2
  Switch5/1 -> Caculate Fault Injected PWM5/2(" Actuator Status[%]")
  Caculate Fault Injected PWM/1(PWM Out) -> [PWM_M1_OUT]
  Caculate Fault Injected PWM1/1(PWM Out) -> [PWM_M2_OUT]
  Caculate Fault Injected PWM2/1(PWM Out) -> [PWM_M3_OUT]
  Caculate Fault Injected PWM3/1(PWM Out) -> [PWM_M4_OUT]
  Caculate Fault Injected PWM4/1(PWM Out) -> [PWM_M5_OUT]
  Caculate Fault Injected PWM5/1(PWM Out) -> [PWM_M6_OUT]

== system MC_HEXA_MISSION/Actuator/Custom Mixer and PWM Output Block/Subsystem ==
  Ch1 : Inport
  Ch2 : Inport  Port=2
  Ch3 : Inport  Port=3
  Ch4 : Inport  Port=4
  Ch5 : Inport  Port=5
  Ch6 : Inport  Port=6
  Bus Assignment : BusAssignment  AssignedSignals=noutputs,output
  Constant : Constant  Value=0
  Constant17 : Constant  Value=6
  Data Type Conversion : DataTypeConversion  OutDataTypeStr=single  SaturateOnIntegerOverflow=off  RndMeth=Floor
  Data Type Conversion1 : DataTypeConversion  OutDataTypeStr=uint32  SaturateOnIntegerOverflow=off  RndMeth=Floor
  Mux1 : Mux  Inputs=16
  PX4 uORB Message : px4uORBlib/PX4 uORB Message  uORBTopic=actuator_outputs  SampleTime=inf  selectInstance=actuator_outputs
  PX4 uORB Write : px4uORBlib/PX4 uORB Write  uORBTopic=actuator_outputs  selectInstance=actuator_outputs  MessageQueueLen=1
  wires:
  Data Type Conversion1/1 -> Bus Assignment/2
  Bus Assignment/1 -> PX4 uORB Write/1
  PX4 uORB Message/1 -> Bus Assignment/1
  Mux1/1 -> Data Type Conversion/1
  Constant17/1 -> Data Type Conversion1/1
  Data Type Conversion/1 -> Bus Assignment/3
  Ch1/1 -> Mux1/1
  Ch2/1 -> Mux1/2
  Ch3/1 -> Mux1/3
  Ch4/1 -> Mux1/4
  Ch5/1 -> Mux1/5
  Ch6/1 -> Mux1/6
  Constant/1 -> Mux1/13, Mux1/14, Mux1/16, Mux1/15, Mux1/12, Mux1/8, Mux1/7, Mux1/9, Mux1/10, Mux1/11

== system MC_HEXA_MISSION/CLAW/Controller/Publish vehicle_attitude_setpoint ==
  note: bX : Body frame ,X axis
  roll_sp : Inport
  pitch_sp : Inport  Port=2
  yaw_sp : Inport  Port=3
  thrust_sp : Inport  Port=4
  Bus Assignment : BusAssignment  AssignedSignals=timestamp,roll_body,pitch_body,yaw_body,thrust_body
  Data Type Conversion{,1..3} (4 alike) : DataTypeConversion  OutDataTypeStr=single  SaturateOnIntegerOverflow=off  RndMeth=Floor
  Mux : Mux  Inputs=3
  PX4 Timestamp : px4Utilslib/PX4 Timestamp  SampleTime=-1
  PX4 uORB Message : px4uORBlib/PX4 uORB Message  uORBTopic=vehicle_attitude_setpoint  SampleTime=-1  selectInstance=actuator_controls
  PX4 uORB Write : px4uORBlib/PX4 uORB Write  uORBTopic=vehicle_attitude_setpoint  selectInstance=vehicle_attitude_setpoint  MessageQueueLen=1
  thrust_sp_bX : Constant  Value=0
  thrust_sp_bY : Constant  Value=0
  wires:
  PX4 Timestamp/1 -> Bus Assignment/2
  Bus Assignment/1 -> PX4 uORB Write/1
  PX4 uORB Message/1 -> Bus Assignment/1
  roll_sp/1 -> Data Type Conversion/1
  pitch_sp/1 -> Data Type Conversion1/1
  yaw_sp/1 -> Data Type Conversion2/1
  Data Type Conversion/1 -> Bus Assignment/3
  Data Type Conversion1/1 -> Bus Assignment/4
  Data Type Conversion2/1 -> Bus Assignment/5
  thrust_sp_bX/1 -> Mux/1
  thrust_sp_bY/1 -> Mux/2
  thrust_sp/1 -> Mux/3
  Mux/1 -> Data Type Conversion3/1
  Data Type Conversion3/1 -> Bus Assignment/6

== system MC_HEXA_MISSION/CLAW/Controller/Publish vehicle_rate_setpoint ==
  note: bX : Body frame ,X axis
  rollrate_sp : Inport
  pitchrate_sp : Inport  Port=2
  yawrate_sp : Inport  Port=3
  thrust_sp : Inport  Port=4
  Bus Assignment : BusAssignment  AssignedSignals=timestamp,roll,pitch,yaw,thrust_body
  Data Type Conversion{,1..3} (4 alike) : DataTypeConversion  OutDataTypeStr=single  SaturateOnIntegerOverflow=off  RndMeth=Floor
  Mux : Mux  Inputs=3
  PX4 Timestamp : px4Utilslib/PX4 Timestamp  SampleTime=-1
  PX4 uORB Message : px4uORBlib/PX4 uORB Message  uORBTopic=vehicle_rates_setpoint  SampleTime=-1  selectInstance=vehicle_rates_setpoint
  PX4 uORB Write : px4uORBlib/PX4 uORB Write  uORBTopic=vehicle_rates_setpoint  selectInstance=vehicle_rates_setpoint  MessageQueueLen=1
  thrust_sp_bX : Constant  Value=0
  thrust_sp_bY : Constant  Value=0
  wires:
  PX4 Timestamp/1 -> Bus Assignment/2
  Bus Assignment/1 -> PX4 uORB Write/1
  PX4 uORB Message/1 -> Bus Assignment/1
  rollrate_sp/1 -> Data Type Conversion/1
  pitchrate_sp/1 -> Data Type Conversion1/1
  yawrate_sp/1 -> Data Type Conversion2/1
  Data Type Conversion/1 -> Bus Assignment/3
  Data Type Conversion1/1 -> Bus Assignment/4
  Data Type Conversion2/1 -> Bus Assignment/5
  thrust_sp_bX/1 -> Mux/1
  thrust_sp_bY/1 -> Mux/2
  thrust_sp/1 -> Mux/3
  Mux/1 -> Data Type Conversion3/1
  Data Type Conversion3/1 -> Bus Assignment/6

== system MC_HEXA_MISSION/CLAW/Controller/Quaternion Validity Check ==
  In1 : Inport
  Constant : Constant  Value=[1 0 0 0]  SampleTime=-1
  Quaternion Norm : sharedutil/Quaternion Norm  aMode=aMode
  Switch : Switch  Criteria=u2 > Threshold  SaturateOnIntegerOverflow=off  InputSameDT=off
  Valid quat : Outport
  wires:
  In1/1 -> Quaternion Norm/1, Switch/1
  Quaternion Norm/1 -> Switch/2
  Switch/1 -> Valid quat/1
  Constant/1 -> Switch/3

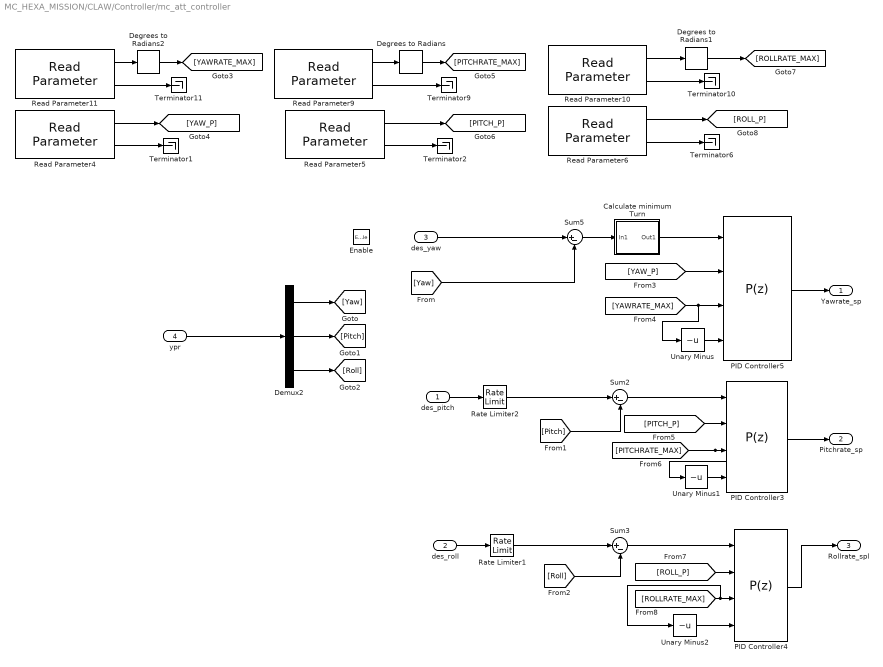
== system MC_HEXA_MISSION/CLAW/Controller/mc_att_controller ==
  des_pitch : Inport
  des_roll : Inport  Port=2
  des_yaw : Inport  Port=3
  ypr : Inport  Port=4
  Enable : EnablePort
  Calculate minimum Turn : Subsystem
  Degrees to Radians : simulink_extras/Transformations/Degrees to Radians
  Degrees to Radians1 : simulink_extras/Transformations/Degrees to Radians
  Degrees to Radians2 : simulink_extras/Transformations/Degrees to Radians
  Demux2 : Demux  Outputs=3
  PID Controller3 : slpidlib/PID Controller  Controller=P  Form=Parallel  TimeDomain=Discrete-time  UseExternalTs=off  SampleTime=-1  IntegratorMethod=Forward Euler  FilterMethod=Forward Euler  ControllerParametersSource=external  P=MC_PITCH_P  I=1  UseKiTs=off  D=0  N=100  UseFilter=on  TunerSelectOption=Transfer Function Based (PID Tuner App)  InitialConditionSource=internal  InitialConditionForIntegrator=0  InitialConditionForFilter=0  DifferentiatorICPrevScaledInput=0  ExternalReset=none  TrackingMode=off  Kt=1  LimitOutput=on  SatLimitsSource=external  UpperSaturationLimit=inf  LowerSaturationLimit=-inf  LinearizeAsGain=on  AntiWindupMode=none  Kb=1  LimitIntegrator=off  UpperIntegratorSaturationLimit=inf  LowerIntegratorSaturationLimit=-inf  POutMin=[]  POutMax=[]  IOutMin=[]  IOutMax=[]  DOutMin=[]  DOutMax=[]  NOutMin=[]  NOutMax=[]  SumOutMin=[]  SumOutMax=[]  SaturationOutMin=[]  SaturationOutMax=[]  PParamMin=[]  PParamMax=[]  IParamMin=[]  IParamMax=[]  DParamMin=[]  DParamMax=[]  NParamMin=[]  NParamMax=[]  KbParamMin=[]  KbParamMax=[]  KtParamMin=[]  KtParamMax=[]  KbOutMin=[]  KbOutMax=[]  KtOutMin=[]  KtOutMax=[]  IntegratorOutMin=[]  IntegratorOutMax=[]  FilterOutMin=[]  FilterOutMax=[]  SumI1OutMin=[]  SumI1OutMax=[]  SumI2OutMin=[]  SumI2OutMax=[]  SumI3OutMin=[]  SumI3OutMax=[]  SumI4OutMin=[]  SumI4OutMax=[]  SumDOutMin=[]  SumDOutMax=[]  DifferentiatorOutMin=[]  DifferentiatorOutMax=[]  FilterDiffOutCoefMin=[]  FilterDiffOutCoefMax=[]  ReciprocalOutMin=[]  ReciprocalOutMax=[]  SumDenOutMin=[]  SumDenOutMax=[]  SumNumOutMin=[]  SumNumOutMax=[]  DivideOutMin=[]  DivideOutMax=[]  UdiffTsProdOutMin=[]  UdiffTsProdOutMax=[]  NTsProdOutMin=[]  NTsProdOutMax=[]  UintegralTsProdOutMin=[]  UintegralTsProdOutMax=[]  UngainTsProdOutMin=[]  UngainTsProdOutMax=[]  ClampingZeroOutDataTypeStr=Inherit: Inherit via back propagation  ClampingZeroOutMin=[]  ClampingZeroOutMax=[]  FilterDenConstantOutDataTypeStr=Inherit: Inherit via back propagation  FilterDenConstantOutMin=[]  FilterDenConstantOutMax=[]  PCopyOutDataTypeStr=Inherit: Inherit via back propagation  PCopyOutMin=[]  PCopyOutMax=[]  NCopyOutDataTypeStr=Inherit: Inherit via back propagation  NCopyOutMin=[]  NCopyOutMax=[]  IntegratorContinuousStateAttributes=''  IntegratorStateMustResolveToSignalObject=off  IntegratorRTWStateStorageClass=Auto  FilterContinuousStateAttributes=''  FilterStateMustResolveToSignalObject=off  FilterRTWStateStorageClass=Auto  ParallelPVariant=ExternalParameters  IdealPVariant=Disabled  IVariant=Disabled  DVariant=Disabled  IntegratorVariant=Disabled  SatVariant=External  AWVariant=Disabled  PCopyVariant=Disabled  TRVariant=Disabled  FdbkBlocksVariant=Forward  IdealPFdbkVariant=Disabled  SatFdbkVariant=Disabled  DerivativeFilterVariant=Disabled  NVariant=Disabled  NCopyVariant=Disabled_SignalSpec  FilterICVariant=Disabled  IntegratorICVariant=Disabled  ExternalResetVariant=Disabled  TRSumVariant=Passthrough  SumFdbkVariant=Disabled  SumVariant=Passthrough_P  TsampFilterVariant=InternalTs  TsampNgainVariant=Passthrough  TsampIntegralVariant=Disabled_SignalSpec  ExternalSaturationOutDataTypeStr=Inherit: Same as second input
  PID Controller4 : slpidlib/PID Controller  Controller=P  Form=Parallel  TimeDomain=Discrete-time  UseExternalTs=off  SampleTime=-1  IntegratorMethod=Forward Euler  FilterMethod=Forward Euler  ControllerParametersSource=external  P=MC_ROLL_P  I=1  UseKiTs=off  D=0  N=100  UseFilter=on  TunerSelectOption=Transfer Function Based (PID Tuner App)  InitialConditionSource=internal  InitialConditionForIntegrator=0  InitialConditionForFilter=0  DifferentiatorICPrevScaledInput=0  ExternalReset=none  TrackingMode=off  Kt=1  LimitOutput=on  SatLimitsSource=external  UpperSaturationLimit=inf  LowerSaturationLimit=-inf  LinearizeAsGain=on  AntiWindupMode=none  Kb=1  LimitIntegrator=off  UpperIntegratorSaturationLimit=inf  LowerIntegratorSaturationLimit=-inf  POutMin=[]  POutMax=[]  IOutMin=[]  IOutMax=[]  DOutMin=[]  DOutMax=[]  NOutMin=[]  NOutMax=[]  SumOutMin=[]  SumOutMax=[]  SaturationOutMin=[]  SaturationOutMax=[]  PParamMin=[]  PParamMax=[]  IParamMin=[]  IParamMax=[]  DParamMin=[]  DParamMax=[]  NParamMin=[]  NParamMax=[]  KbParamMin=[]  KbParamMax=[]  KtParamMin=[]  KtParamMax=[]  KbOutMin=[]  KbOutMax=[]  KtOutMin=[]  KtOutMax=[]  IntegratorOutMin=[]  IntegratorOutMax=[]  FilterOutMin=[]  FilterOutMax=[]  SumI1OutMin=[]  SumI1OutMax=[]  SumI2OutMin=[]  SumI2OutMax=[]  SumI3OutMin=[]  SumI3OutMax=[]  SumI4OutMin=[]  SumI4OutMax=[]  SumDOutMin=[]  SumDOutMax=[]  DifferentiatorOutMin=[]  DifferentiatorOutMax=[]  FilterDiffOutCoefMin=[]  FilterDiffOutCoefMax=[]  ReciprocalOutMin=[]  ReciprocalOutMax=[]  SumDenOutMin=[]  SumDenOutMax=[]  SumNumOutMin=[]  SumNumOutMax=[]  DivideOutMin=[]  DivideOutMax=[]  UdiffTsProdOutMin=[]  UdiffTsProdOutMax=[]  NTsProdOutMin=[]  NTsProdOutMax=[]  UintegralTsProdOutMin=[]  UintegralTsProdOutMax=[]  UngainTsProdOutMin=[]  UngainTsProdOutMax=[]  ClampingZeroOutDataTypeStr=Inherit: Inherit via back propagation  ClampingZeroOutMin=[]  ClampingZeroOutMax=[]  FilterDenConstantOutDataTypeStr=Inherit: Inherit via back propagation  FilterDenConstantOutMin=[]  FilterDenConstantOutMax=[]  PCopyOutDataTypeStr=Inherit: Inherit via back propagation  PCopyOutMin=[]  PCopyOutMax=[]  NCopyOutDataTypeStr=Inherit: Inherit via back propagation  NCopyOutMin=[]  NCopyOutMax=[]  IntegratorContinuousStateAttributes=''  IntegratorStateMustResolveToSignalObject=off  IntegratorRTWStateStorageClass=Auto  FilterContinuousStateAttributes=''  FilterStateMustResolveToSignalObject=off  FilterRTWStateStorageClass=Auto  ParallelPVariant=ExternalParameters  IdealPVariant=Disabled  IVariant=Disabled  DVariant=Disabled  IntegratorVariant=Disabled  SatVariant=External  AWVariant=Disabled  PCopyVariant=Disabled  TRVariant=Disabled  FdbkBlocksVariant=Forward  IdealPFdbkVariant=Disabled  SatFdbkVariant=Disabled  DerivativeFilterVariant=Disabled  NVariant=Disabled  NCopyVariant=Disabled_SignalSpec  FilterICVariant=Disabled  IntegratorICVariant=Disabled  ExternalResetVariant=Disabled  TRSumVariant=Passthrough  SumFdbkVariant=Disabled  SumVariant=Passthrough_P  TsampFilterVariant=InternalTs  TsampNgainVariant=Passthrough  TsampIntegralVariant=Disabled_SignalSpec  ExternalSaturationOutDataTypeStr=Inherit: Same as second input
  PID Controller5 : slpidlib/PID Controller  Controller=P  Form=Parallel  TimeDomain=Discrete-time  UseExternalTs=off  SampleTime=-1  IntegratorMethod=Forward Euler  FilterMethod=Forward Euler  ControllerParametersSource=external  P=MC_YAW_P  I=1  UseKiTs=off  D=0  N=100  UseFilter=on  TunerSelectOption=Transfer Function Based (PID Tuner App)  InitialConditionSource=internal  InitialConditionForIntegrator=0  InitialConditionForFilter=0  DifferentiatorICPrevScaledInput=0  ExternalReset=none  TrackingMode=off  Kt=1  LimitOutput=on  SatLimitsSource=external  UpperSaturationLimit=50*pi/180  LowerSaturationLimit=-50*pi/180  LinearizeAsGain=on  AntiWindupMode=none  Kb=1  LimitIntegrator=off  UpperIntegratorSaturationLimit=inf  LowerIntegratorSaturationLimit=-inf  POutMin=[]  POutMax=[]  IOutMin=[]  IOutMax=[]  DOutMin=[]  DOutMax=[]  NOutMin=[]  NOutMax=[]  SumOutMin=[]  SumOutMax=[]  SaturationOutMin=[]  SaturationOutMax=[]  PParamMin=[]  PParamMax=[]  IParamMin=[]  IParamMax=[]  DParamMin=[]  DParamMax=[]  NParamMin=[]  NParamMax=[]  KbParamMin=[]  KbParamMax=[]  KtParamMin=[]  KtParamMax=[]  KbOutMin=[]  KbOutMax=[]  KtOutMin=[]  KtOutMax=[]  IntegratorOutMin=[]  IntegratorOutMax=[]  FilterOutMin=[]  FilterOutMax=[]  SumI1OutMin=[]  SumI1OutMax=[]  SumI2OutMin=[]  SumI2OutMax=[]  SumI3OutMin=[]  SumI3OutMax=[]  SumI4OutMin=[]  SumI4OutMax=[]  SumDOutMin=[]  SumDOutMax=[]  DifferentiatorOutMin=[]  DifferentiatorOutMax=[]  FilterDiffOutCoefMin=[]  FilterDiffOutCoefMax=[]  ReciprocalOutMin=[]  ReciprocalOutMax=[]  SumDenOutMin=[]  SumDenOutMax=[]  SumNumOutMin=[]  SumNumOutMax=[]  DivideOutMin=[]  DivideOutMax=[]  UdiffTsProdOutMin=[]  UdiffTsProdOutMax=[]  NTsProdOutMin=[]  NTsProdOutMax=[]  UintegralTsProdOutMin=[]  UintegralTsProdOutMax=[]  UngainTsProdOutMin=[]  UngainTsProdOutMax=[]  ClampingZeroOutDataTypeStr=Inherit: Inherit via back propagation  ClampingZeroOutMin=[]  ClampingZeroOutMax=[]  FilterDenConstantOutDataTypeStr=Inherit: Inherit via back propagation  FilterDenConstantOutMin=[]  FilterDenConstantOutMax=[]  PCopyOutDataTypeStr=Inherit: Inherit via back propagation  PCopyOutMin=[]  PCopyOutMax=[]  NCopyOutDataTypeStr=Inherit: Inherit via back propagation  NCopyOutMin=[]  NCopyOutMax=[]  IntegratorContinuousStateAttributes=''  IntegratorStateMustResolveToSignalObject=off  IntegratorRTWStateStorageClass=Auto  FilterContinuousStateAttributes=''  FilterStateMustResolveToSignalObject=off  FilterRTWStateStorageClass=Auto  ParallelPVariant=ExternalParameters  IdealPVariant=Disabled  IVariant=Disabled  DVariant=Disabled  IntegratorVariant=Disabled  SatVariant=External  AWVariant=Disabled  PCopyVariant=Disabled  TRVariant=Disabled  FdbkBlocksVariant=Forward  IdealPFdbkVariant=Disabled  SatFdbkVariant=Disabled  DerivativeFilterVariant=Disabled  NVariant=Disabled  NCopyVariant=Disabled_SignalSpec  FilterICVariant=Disabled  IntegratorICVariant=Disabled  ExternalResetVariant=Disabled  TRSumVariant=Passthrough  SumFdbkVariant=Disabled  SumVariant=Passthrough_P  TsampFilterVariant=InternalTs  TsampNgainVariant=Passthrough  TsampIntegralVariant=Disabled_SignalSpec  ExternalSaturationOutDataTypeStr=Inherit: Same as second input
  Rate Limiter1 : RateLimiter  RisingSlewLimit=180*pi/180  FallingSlewLimit=-180*pi/180  SampleTimeMode=inherited
  Rate Limiter2 : RateLimiter  RisingSlewLimit=180*pi/180  FallingSlewLimit=-180*pi/180  SampleTimeMode=inherited
  Read Parameter10 : px4lib/Read Parameter  ParameterName=SL_ROLLRATE_MAX  DataType=FLOAT  SampleTime=-1
  Read Parameter11 : px4lib/Read Parameter  ParameterName=SL_YAWRATE_MAX  DataType=FLOAT  SampleTime=-1
  Read Parameter4 : px4lib/Read Parameter  ParameterName=SL_YAW_P  DataType=FLOAT  SampleTime=-1
  Read Parameter5 : px4lib/Read Parameter  ParameterName=SL_PITCH_P  DataType=FLOAT  SampleTime=-1
  Read Parameter6 : px4lib/Read Parameter  ParameterName=SL_ROLL_P  DataType=FLOAT  SampleTime=-1
  Read Parameter9 : px4lib/Read Parameter  ParameterName=SL_PITCHRATE_MAX  DataType=FLOAT  SampleTime=-1
  Sum2 : Sum  Inputs=|+-
  Sum3 : Sum  Inputs=|+-
  Sum5 : Sum  Inputs=|+-
  Terminator{1..2,6,9..11} (6 alike) : Terminator
  Unary Minus : UnaryMinus
  Unary Minus1 : UnaryMinus
  Unary Minus2 : UnaryMinus
  Yawrate_sp : Outport
  Pitchrate_sp : Outport  Port=2
  Rollrate_spl : Outport  Port=3
  wires:
  Sum2/1 -> PID Controller3/1
  Sum3/1 -> PID Controller4/1
  ypr/1 -> Demux2/1
  Sum5/1 -> Calculate minimum Turn/1(In1)
  Calculate minimum Turn/1(Out1) -> PID Controller5/1
  des_roll/1 -> Rate Limiter1/1
  des_yaw/1 -> Sum5/1
  Rate Limiter1/1 -> Sum3/1
  Rate Limiter2/1 -> Sum2/1
  des_pitch/1 -> Rate Limiter2/1
  PID Controller5/1 -> Yawrate_sp/1
  PID Controller3/1 -> Pitchrate_sp/1
  PID Controller4/1 -> Rollrate_spl/1
  Demux2/1 -> [Yaw]
  Demux2/2 -> [Pitch]
  Demux2/3 -> [Roll]
  [Yaw] -> Sum5/2
  [Pitch] -> Sum2/2
  [Roll] -> Sum3/2
  Read Parameter6/1 -> [ROLL_P]
  Read Parameter4/1 -> [YAW_P]
  Read Parameter5/1 -> [PITCH_P]
  Read Parameter10/2 -> Terminator10/1
  Read Parameter11/1 -> Degrees to Radians2/1
  Read Parameter11/2 -> Terminator11/1
  Read Parameter9/2 -> Terminator9/1
  Read Parameter10/1 -> Degrees to Radians1/1
  Read Parameter9/1 -> Degrees to Radians/1
  Read Parameter4/2 -> Terminator1/1
  Read Parameter5/2 -> Terminator2/1
  Read Parameter6/2 -> Terminator6/1
  [YAW_P] -> PID Controller5/2
  [YAWRATE_MAX] -> Unary Minus/1, PID Controller5/3
  Unary Minus/1 -> PID Controller5/4
  [PITCH_P] -> PID Controller3/2
  [PITCHRATE_MAX] -> Unary Minus1/1, PID Controller3/3
  Unary Minus1/1 -> PID Controller3/4
  [ROLL_P] -> PID Controller4/2
  [ROLLRATE_MAX] -> Unary Minus2/1, PID Controller4/3
  Unary Minus2/1 -> PID Controller4/4
  Degrees to Radians1/1 -> [ROLLRATE_MAX]
  Degrees to Radians/1 -> [PITCHRATE_MAX]
  Degrees to Radians2/1 -> [YAWRATE_MAX]
